simulink library "lib_temperature_compensator"  (R2023a)
settings: Solver=VariableStepAuto  StartTime=0.0  StopTime=10.0  RelTol=1e-3
settings Model: Creator=cav2ofo  LastModifiedBy=lenovo
settings OptimizationCC: ReuseModelBlockBuffer=off

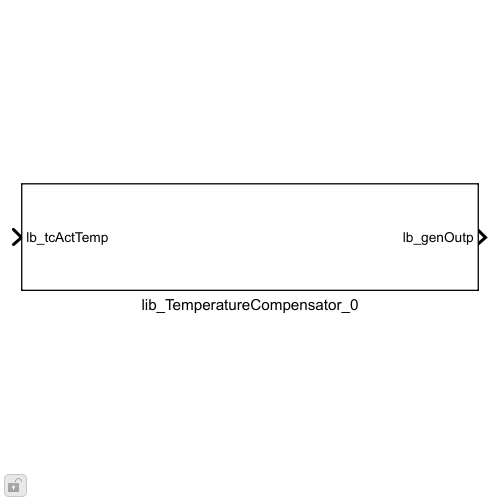
[thumbnail: Simulink's stored preview of the top-level diagram]
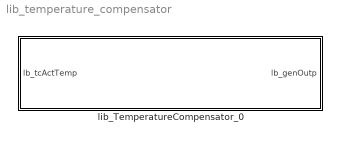
== system lib_temperature_compensator ==
  lib_TemperatureCompensator_0 : Subsystem  mask{lb_parTempCoef=-1e-3, lb_parRefTemp=20, lb_parRefTempOutpVal=0}
      mask prompts: lb_parTempCoef "Temperature coefficient [1/K]:"; lb_parRefTemp "Reference temperature [oC]:"; lb_parRefTempOutpVal "Output value at reference temperature [ou]:"
      mask DialogControl DescGroupVar Prompt: VHIT control library
      mask DialogControl DescTextVar Prompt: Temperature compensator

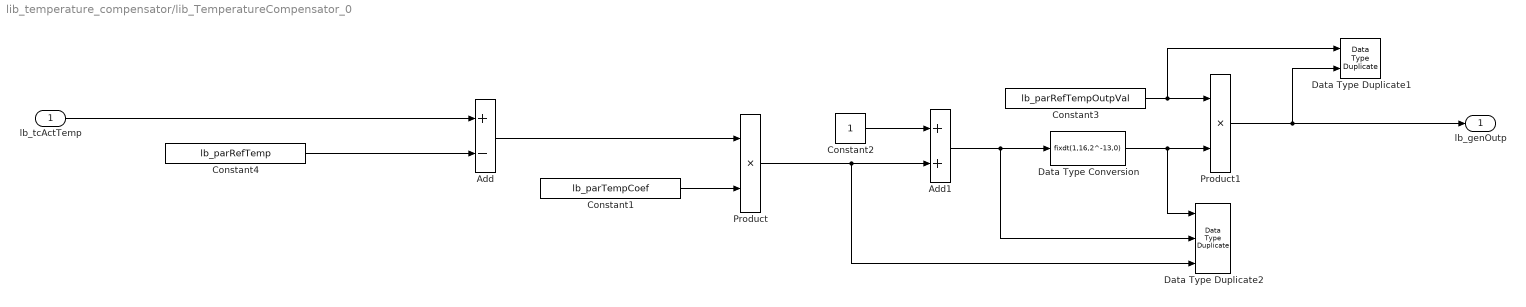
== system lib_temperature_compensator/lib_TemperatureCompensator_0 ==
  lb_tcActTemp : Inport
  Add : Sum  Inputs=+-  OutDataTypeStr=Inherit: Same as first input
  Add1 : Sum  OutDataTypeStr=Inherit: Inherit via back propagation
  Constant1 : Constant  Value=lb_parTempCoef
  Constant2 : Constant  OutDataTypeStr=uint8
  Constant3 : Constant  Value=lb_parRefTempOutpVal
  Constant4 : Constant  Value=lb_parRefTemp
  Data Type Duplicate1 : DataTypeDuplicate
  Data Type Duplicate2 : DataTypeDuplicate  NumInputPorts=3
  Data Type Conversion : DataTypeConversion  OutDataTypeStr=fixdt(1,16,2^-13,0)  SaturateOnIntegerOverflow=off  RndMeth=Floor
  Product : Product  OutDataTypeStr=Inherit: Inherit via back propagation
  Product1 : Product  OutDataTypeStr=Inherit: Inherit via back propagation
  lb_genOutp : Outport  VectorParamsAs1DForOutWhenUnconnected=off
  wires:
  Product1/1 -> Data Type Duplicate1/2, lb_genOutp/1
  lb_tcActTemp/1 -> Add/1
  Constant4/1 -> Add/2
  Add/1 -> Product/1
  Constant1/1 -> Product/2
  Product/1 -> Data Type Duplicate2/3, Add1/2
  Constant2/1 -> Add1/1
  Add1/1 -> Data Type Conversion/1, Data Type Duplicate2/2
  Constant3/1 -> Data Type Duplicate1/1, Product1/1
  Data Type Conversion/1 -> Data Type Duplicate2/1, Product1/2
